simulink model "state_estimator"  (R2025b)
settings: Solver=VariableStepAuto  StartTime=0.0  StopTime=10.0  RelTol=1e-3
settings Model: LastModifiedBy=jak64

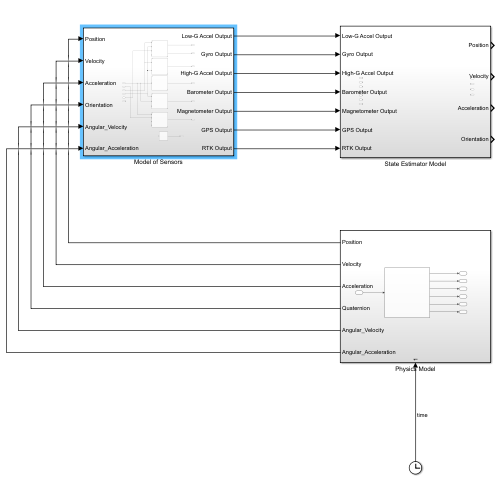
[thumbnail: Simulink's stored preview of the top-level diagram]
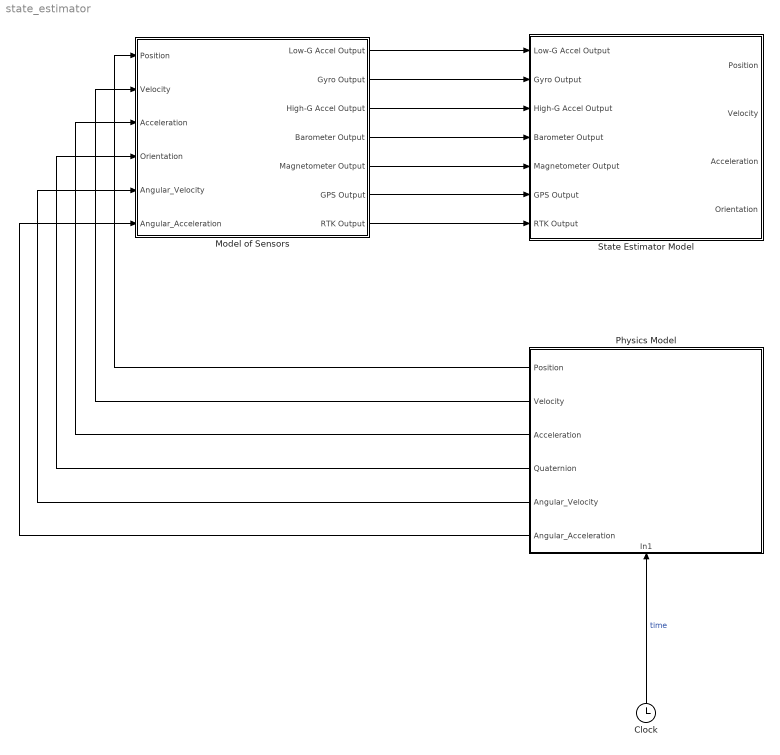
== system state_estimator ==
  Clock : Clock
  Model of Sensors : Subsystem
  Physics Model : Subsystem
      settings: PortSchema="{\"entries\":[{\"content\":{\"sides\":[{\"content\":{\"connectorIds\":[\"Out1\",\"Out2\",\"Out3\",\"Out4\",\"Out5\",\"Out6\"]},\"type\":\"ConnectorPlacement.EquallySpacedRectSide\",\"uuid\":\"d973089c-7b51-4721-858e-49b2da9ba2e2\"},{\"content\":{\"side\":\"RIGHT\"},\"type\":\"ConnectorPlacement.EquallySpacedRectSide\",\"uuid\":\"a0a62891-f020-44a5-9f44-1534f6d7597c\"},{\"content\":{\"side\":\"TOP\"},\"type\":\"ConnectorPlacement.EquallySpacedRectSide\",\"uuid\":\"420ffd3e-2259-443b-b734-66425db33e5d\"},{\"content\":{\"connectorIds\":[\"In1\"],\"side\":\"BOTTOM\"},\"type\":\"ConnectorPlacement.EquallySpacedRectSide\",\"uuid\":\"61b4c197-8443-47ca-8602-966eda63e0fb\"}]},\"type\":\"ConnectorPlacement.EquallySpacedConnector\",\"uuid\":\"7be80f26-ca88-418d-b859-dfd10cd1bf87\"}],\"packageUris\":[\"http://schema.mathworks.com/mf0/Connector/R2020b\"],\"version\":\"1.0\"}"
  State Estimator Model : Subsystem
  wires:
  Clock/1 -> Physics Model/1(In1)  "time"
  Physics Model/1(Position) -> Model of Sensors/1(Position)
  Physics Model/2(Velocity) -> Model of Sensors/2(Velocity)
  Physics Model/3(Acceleration) -> Model of Sensors/3(Acceleration)
  Physics Model/4(Quaternion) -> Model of Sensors/4(Orientation)
  Model of Sensors/1(Low-G Accel Output) -> State Estimator Model/1(Low-G Accel Output)
  Model of Sensors/3(High-G Accel Output) -> State Estimator Model/3(High-G Accel Output)
  Model of Sensors/4(Barometer Output) -> State Estimator Model/4(Barometer Output)
  Model of Sensors/5(Magnetometer Output) -> State Estimator Model/5(Magnetometer Output)
  Model of Sensors/6(GPS Output) -> State Estimator Model/6(GPS Output)
  Model of Sensors/7(RTK Output) -> State Estimator Model/7(RTK Output)
  Model of Sensors/2(Gyro Output) -> State Estimator Model/2(Gyro Output)
  Physics Model/5(Angular_Velocity) -> Model of Sensors/5(Angular_Velocity)
  Physics Model/6(Angular_Acceleration) -> Model of Sensors/6(Angular_Acceleration)

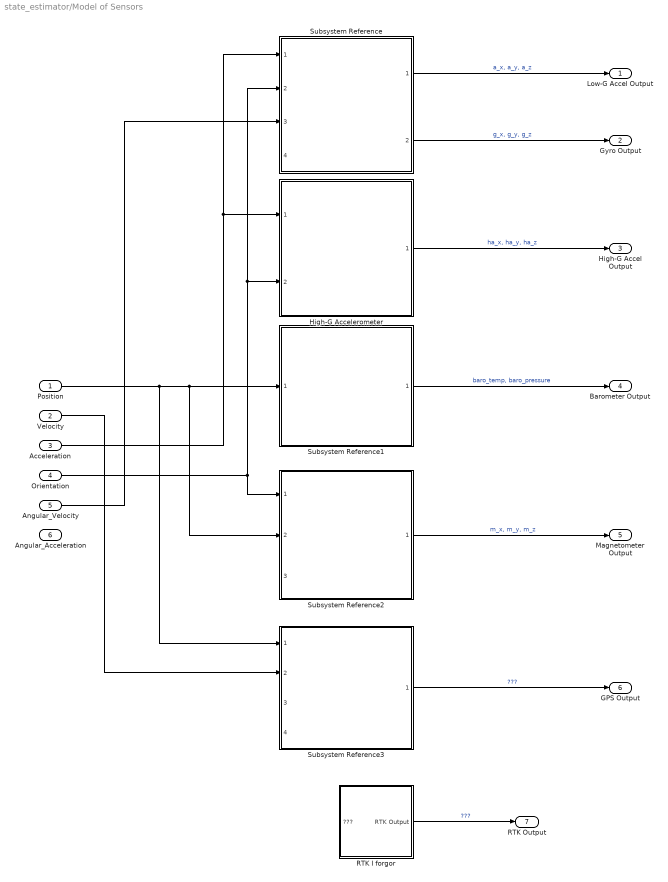
== system state_estimator/Model of Sensors ==
  Position : Inport
  Velocity : Inport  Port=2
  Acceleration : Inport  Port=3
  Orientation : Inport  Port=4
  Angular_Velocity : Inport  Port=5
  Angular_Acceleration : Inport  Port=6
  "High-G Accelerometer " : Subsystem  ReferencedSubsystem=H3LIS331DLTR
  RTK I forgor : Subsystem
  Subsystem Reference : Subsystem  ReferencedSubsystem=ICM_20608_G
  Subsystem Reference1 : Subsystem  ReferencedSubsystem=Barometer_DPS368
  Subsystem Reference2 : Subsystem  ReferencedSubsystem=Magnetometer_MMC5983MA
  Subsystem Reference3 : Subsystem  ReferencedSubsystem=GPS_MAX_M10S
  Low-G Accel Output : Outport
  Gyro Output : Outport  Port=2
  High-G Accel Output : Outport  Port=3
  Barometer Output : Outport  Port=4
  Magnetometer Output : Outport  Port=5
  GPS Output : Outport  Port=6
  RTK Output : Outport  Port=7
  wires:
  Orientation/1 -> Subsystem Reference2/1, Subsystem Reference/2, "High-G Accelerometer "/2
  "High-G Accelerometer "/1 -> High-G Accel Output/1  "ha_x, ha_y, ha_z"
  Subsystem Reference/1 -> Low-G Accel Output/1  "a_x, a_y, a_z"
  Subsystem Reference/2 -> Gyro Output/1  "g_x, g_y, g_z"
  Acceleration/1 -> Subsystem Reference/1, "High-G Accelerometer "/1
  Angular_Velocity/1 -> Subsystem Reference/3
  Subsystem Reference1/1 -> Barometer Output/1  "baro_temp, baro_pressure"
  Subsystem Reference2/1 -> Magnetometer Output/1  "m_x, m_y, m_z"
  Subsystem Reference3/1 -> GPS Output/1  "???"
  RTK I forgor/1(RTK Output) -> RTK Output/1  "???"
  Position/1 -> Subsystem Reference3/1, Subsystem Reference2/2, Subsystem Reference1/1
  Velocity/1 -> Subsystem Reference3/2

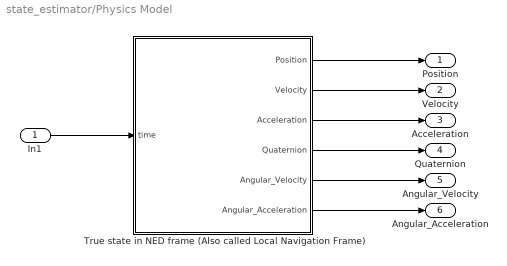
== system state_estimator/Physics Model ==
  In1 : Inport
  True state in NED frame (Also called Local Navigation Frame) : MATLAB Function  TreatAsAtomicUnit=on
  Position : Outport
  Velocity : Outport  Port=2
  Acceleration : Outport  Port=3
  Quaternion : Outport  Port=4
  Angular_Velocity : Outport  Port=5
  Angular_Acceleration : Outport  Port=6
  wires:
  In1/1 -> True state in NED frame (Also called Local Navigation Frame)/1(time)
  True state in NED frame (Also called Local Navigation Frame)/4(Quaternion) -> Quaternion/1
  True state in NED frame (Also called Local Navigation Frame)/2(Velocity) -> Velocity/1
  True state in NED frame (Also called Local Navigation Frame)/1(Position) -> Position/1
  True state in NED frame (Also called Local Navigation Frame)/3(Acceleration) -> Acceleration/1
  True state in NED frame (Also called Local Navigation Frame)/5(Angular_Velocity) -> Angular_Velocity/1
  True state in NED frame (Also called Local Navigation Frame)/6(Angular_Acceleration) -> Angular_Acceleration/1

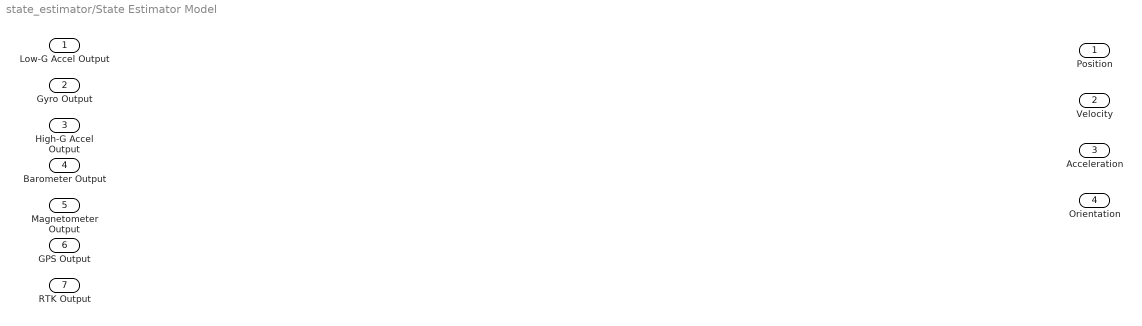
== system state_estimator/State Estimator Model ==
  Low-G Accel Output : Inport
  Gyro Output : Inport  Port=2
  High-G Accel Output : Inport  Port=3
  Barometer Output : Inport  Port=4
  Magnetometer Output : Inport  Port=5
  GPS Output : Inport  Port=6
  RTK Output : Inport  Port=7
  Position : Outport
  Velocity : Outport  Port=2
  Acceleration : Outport  Port=3
  Orientation : Outport  Port=4

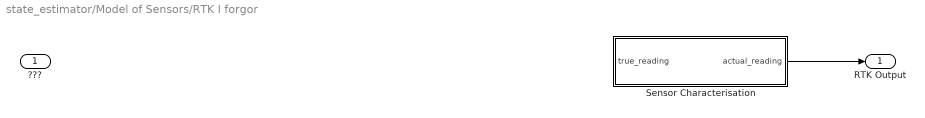
== system state_estimator/Model of Sensors/RTK I forgor ==
  "???" : Inport
  Sensor Characterisation : MATLAB Function  TreatAsAtomicUnit=on
  RTK Output : Outport
  wires:
  Sensor Characterisation/1(actual_reading) -> RTK Output/1
  ? -> Sensor Characterisation/1(true_reading)  "state"

== matlab function state_estimator/Physics Model/True state in NED frame (Also called Local Navigation Frame) ==
  data: time input; Position output; Velocity output; Acceleration output; Quaternion output; Angular_Velocity output; Angular_Acceleration output
function [Position, Velocity, Acceleration, Quaternion, Angular_Velocity, Angular_Acceleration] = fcn(time)

% --- EKF states ---
Position  = [0; 0; 0];       % m
Velocity  = [0; 0; 0];       % m/s

Quaternion = [1; 0; 0; 0];    % unit quaternion (no rotation)
Angular_Velocity = [0; 0; 0]; % rad/s

% --- Sensor measured states ---
Acceleration  = [0; 0; 0];       % m/s^2
Angular_Acceleration = [0; 0; 0]; % rad/s^2
end

== matlab function state_estimator/Model of Sensors/RTK I forgor/Sensor Characterisation ==
  data: true_reading input; actual_reading output
function actual_reading = fcn(true_reading)
    persistent b_previous

    dt = 0.0553; % Simulation Time Step[s]

    % Bias: Composite Bias = Const + Gauss-Markov Drift
    
        b_const = [-7.395250; -4.820243; -18.177021]; % Constant bias
    
        % Drift bias (b = exp^-dt/tau * b_previous + omega)
        
        if isempty(b_previous)
            b_previous = [0 0 0]; 
        end
    
        tau = [8.731; 8.731; 8.731]; % time constant of drift
        q = [8.774166e-04; 7.720775e-04; 1.336849e-03]; % variance on drift
    
        omega = sqrt(q) .* randn(3,1); % omega ~ N(0,q)
        
        b_drift = exp(-dt ./ tau) .* b_previous + omega;
    
        composite_bias = b_const + b_drift; 

    % Noise: Gaussian  

        noise_variance = [1.645664; 1.487596; 1.836378]; 
    
        noise = noise_variance .* randn(3,1); 
    
    % Quantisation:

        quant_step = 0.5; % Quant Step: data sheet
   

    % Reading Processing:

        actual_reading_continuous  = true_reading(:) + composite_bias + noise;

        actual_reading_quantised = quant_step * round(actual_reading_continuous/quant_step);

        actual_reading = actual_reading_quantised; 

end

% Currently Ignoring: 
% Scale_factor_error 
% Misalignment_error
